simulink model "EPT"  (R2019b)
settings: Solver=FixedStepDiscrete  StartTime=0.0  StopTime=5  FixedStep=0.005  RelTol=1e-3  EnableMultiTasking=on
PreLoadFcn:
  | try, model_open; catch, disp('Error occurred while executing model pre-load callback: model_open.m'); disp('Please assure that the MATLAB working directory is set to the model directory before opening.'); end
InitFcn:
  | try, model_open; catch, end
undefined symbols (not defined in the file or in its folder): Bridge, GCM, H, ln, raptor_get_param_eval, raptor_get_safe_string, raptor_xcp_function
libraries: Raptor_lib x2810, simulink x374, hdlsllib x19
(part 24 of 45)

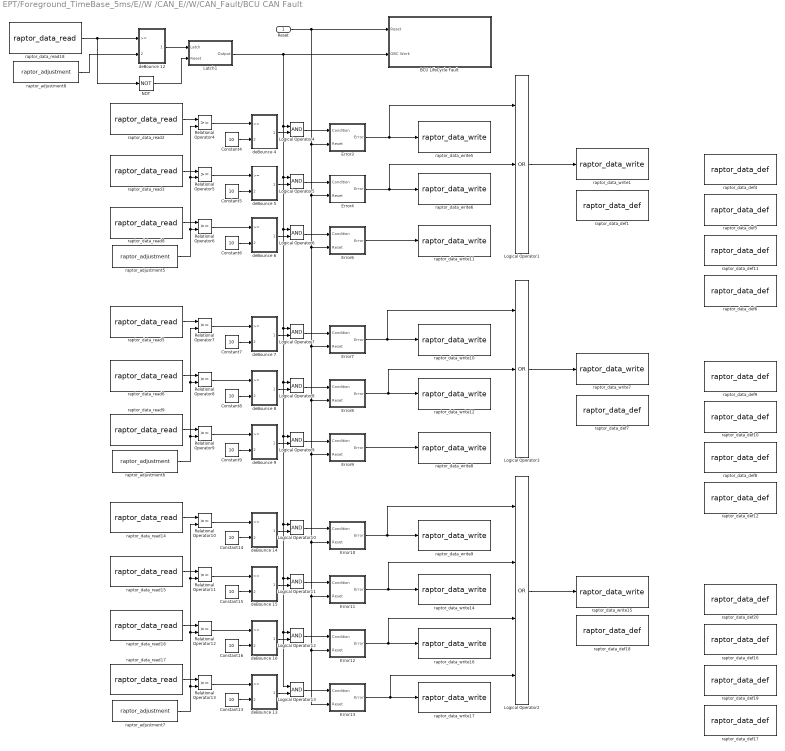
== system EPT/Foreground_TimeBase_5ms/E//W /CAN_E//W/CAN_Fault/BCU CAN Fault ==
  Reset : Inport
  BCU LifeCycle Fault : Subsystem
  Constant{4..9,13..16} (10 alike) : Constant  Value=10
  Error10 : Subsystem
  Error11 : Subsystem
  Error12 : Subsystem
  Error13 : Subsystem
  Error3 : Subsystem
  Error4 : Subsystem
  Error6 : Subsystem
  Error7 : Subsystem
  Error8 : Subsystem
  Error9 : Subsystem
  Latch1 : Subsystem
  Logical Operator1 : Logic  Operator=OR  Inputs=3  AllPortsSameDT=off  OutDataTypeStr=boolean
  Logical Operator{4..13} (10 alike) : Logic  AllPortsSameDT=off  OutDataTypeStr=boolean
  Logical Operator2 : Logic  Operator=OR  Inputs=4  AllPortsSameDT=off  OutDataTypeStr=boolean
  Logical Operator3 : Logic  Operator=OR  Inputs=3  AllPortsSameDT=off  OutDataTypeStr=boolean
  NOT : Logic  Operator=NOT  IconShape=distinctive  AllPortsSameDT=off  OutDataTypeStr=boolean
  Relational Operator{4..13} (10 alike) : RelationalOperator  OutDataTypeStr=boolean  RndMeth=Simplest
  deBounce 12 : Subsystem
  deBounce 13 : Subsystem
  deBounce 14 : Subsystem
  deBounce 15 : Subsystem
  deBounce 16 : Subsystem
  deBounce 4 : Subsystem
  deBounce 5 : Subsystem
  deBounce 6 : Subsystem
  deBounce 7 : Subsystem
  deBounce 8 : Subsystem
  deBounce 9 : Subsystem
  raptor_adjustment5 : Raptor_lib/Data Storage/raptor_adjustment  paramName='CMU1_Age_Time'  nameSource=Parameter  initValue=5  dataType=uint16  storage=Calibration  calDispType=Number  calEnum={'False', 'True'}  calGain=1.0  calOffset=0.0  calMax=inf  calMin=-inf  calFormat='-1'  calUnit=''  calHelp=''  calAccess=1  calFunction=raptor_xcp_function(gcb)  calDispHeaders=off  calColHeaders={'Col1' 'Col2' 'Col3'}  calRowHeaders={'Row1' 'Row2' 'Row3'}
      settings: SourceProductName=Raptor
  raptor_adjustment6 : Raptor_lib/Data Storage/raptor_adjustment  paramName='CMU2_Age_Time'  nameSource=Parameter  initValue=5  dataType=uint16  storage=Calibration  calDispType=Number  calEnum={'False', 'True'}  calGain=1.0  calOffset=0.0  calMax=inf  calMin=-inf  calFormat='-1'  calUnit=''  calHelp=''  calAccess=1  calFunction=raptor_xcp_function(gcb)  calDispHeaders=off  calColHeaders={'Col1' 'Col2' 'Col3'}  calRowHeaders={'Row1' 'Row2' 'Row3'}
      settings: SourceProductName=Raptor
  raptor_adjustment7 : Raptor_lib/Data Storage/raptor_adjustment  paramName='IVT_Age_Time'  nameSource=Parameter  initValue=5  dataType=uint16  storage=Calibration  calDispType=Number  calEnum={'False', 'True'}  calGain=1.0  calOffset=0.0  calMax=inf  calMin=-inf  calFormat='-1'  calUnit=''  calHelp=''  calAccess=1  calFunction=raptor_xcp_function(gcb)  calDispHeaders=off  calColHeaders={'Col1' 'Col2' 'Col3'}  calRowHeaders={'Row1' 'Row2' 'Row3'}
      settings: SourceProductName=Raptor
  raptor_adjustment8 : Raptor_lib/Data Storage/raptor_adjustment  paramName='Cal_BCU_CANFault_TimeCount'  nameSource=Parameter  initValue=300  dataType=double  storage=Calibration  calDispType=Number  calEnum={'False', 'True'}  calGain=1.0  calOffset=0.0  calMax=inf  calMin=-inf  calFormat='-1'  calUnit=''  calHelp=''  calAccess=1  calFunction=raptor_xcp_function(gcb)  calDispHeaders=off  calColHeaders={'Col1' 'Col2' 'Col3'}  calRowHeaders={'Row1' 'Row2' 'Row3'}
      settings: SourceProductName=Raptor
  raptor_data_def1 : Raptor_lib/Data Storage/raptor_data_def  dataName='CAN_Fault_CMU1'  initValue=0  dataType=boolean  storage=Volatile (RAM)  calVisible=on  calType=Measurement  calDispType=Number  calEnum={'False', 'True'}  calGain=1.0  calOffset=0  calMin=-inf  calMax=inf  calFormat='-1'  calUnit=''  calHelp=''  calAccess=1  calFunction=raptor_xcp_function(gcb)  calDispHeaders=off  calColHeaders={'Col1' 'Col2' 'Col3'}  calRowHeaders={'Row1' 'Row2' 'Row3'}
      settings: SourceProductName=Raptor
  raptor_data_def10 : Raptor_lib/Data Storage/raptor_data_def  dataName='CAN_Fault_CMU200B1A2'  initValue=0  dataType=boolean  storage=Volatile (RAM)  calVisible=on  calType=Measurement  calDispType=Number  calEnum={'False', 'True'}  calGain=1.0  calOffset=0  calMin=-inf  calMax=inf  calFormat='-1'  calUnit=''  calHelp=''  calAccess=1  calFunction=raptor_xcp_function(gcb)  calDispHeaders=off  calColHeaders={'Col1' 'Col2' 'Col3'}  calRowHeaders={'Row1' 'Row2' 'Row3'}
      settings: SourceProductName=Raptor
  raptor_data_def11 : Raptor_lib/Data Storage/raptor_data_def  dataName='CAN_Fault_CMU200B2A1'  initValue=0  dataType=boolean  storage=Volatile (RAM)  calVisible=on  calType=Measurement  calDispType=Number  calEnum={'False', 'True'}  calGain=1.0  calOffset=0  calMin=-inf  calMax=inf  calFormat='-1'  calUnit=''  calHelp=''  calAccess=1  calFunction=raptor_xcp_function(gcb)  calDispHeaders=off  calColHeaders={'Col1' 'Col2' 'Col3'}  calRowHeaders={'Row1' 'Row2' 'Row3'}
      settings: SourceProductName=Raptor
  raptor_data_def12 : Raptor_lib/Data Storage/raptor_data_def  dataName='CAN_Fault_CMU200BAA2'  initValue=0  dataType=boolean  storage=Volatile (RAM)  calVisible=on  calType=Measurement  calDispType=Number  calEnum={'False', 'True'}  calGain=1.0  calOffset=0  calMin=-inf  calMax=inf  calFormat='-1'  calUnit=''  calHelp=''  calAccess=1  calFunction=raptor_xcp_function(gcb)  calDispHeaders=off  calColHeaders={'Col1' 'Col2' 'Col3'}  calRowHeaders={'Row1' 'Row2' 'Row3'}
      settings: SourceProductName=Raptor
  raptor_data_def16 : Raptor_lib/Data Storage/raptor_data_def  dataName='CAN_Fault_0x522'  initValue=0  dataType=boolean  storage=Volatile (RAM)  calVisible=on  calType=Measurement  calDispType=Number  calEnum={'False', 'True'}  calGain=1.0  calOffset=0  calMin=-inf  calMax=inf  calFormat='-1'  calUnit=''  calHelp=''  calAccess=1  calFunction=raptor_xcp_function(gcb)  calDispHeaders=off  calColHeaders={'Col1' 'Col2' 'Col3'}  calRowHeaders={'Row1' 'Row2' 'Row3'}
      settings: SourceProductName=Raptor
  raptor_data_def17 : Raptor_lib/Data Storage/raptor_data_def  dataName='CAN_Fault_0x524'  initValue=0  dataType=boolean  storage=Volatile (RAM)  calVisible=on  calType=Measurement  calDispType=Number  calEnum={'False', 'True'}  calGain=1.0  calOffset=0  calMin=-inf  calMax=inf  calFormat='-1'  calUnit=''  calHelp=''  calAccess=1  calFunction=raptor_xcp_function(gcb)  calDispHeaders=off  calColHeaders={'Col1' 'Col2' 'Col3'}  calRowHeaders={'Row1' 'Row2' 'Row3'}
      settings: SourceProductName=Raptor
  raptor_data_def18 : Raptor_lib/Data Storage/raptor_data_def  dataName='CAN_Fault_IVT'  initValue=0  dataType=boolean  storage=Volatile (RAM)  calVisible=on  calType=Measurement  calDispType=Number  calEnum={'False', 'True'}  calGain=1.0  calOffset=0  calMin=-inf  calMax=inf  calFormat='-1'  calUnit=''  calHelp=''  calAccess=1  calFunction=raptor_xcp_function(gcb)  calDispHeaders=off  calColHeaders={'Col1' 'Col2' 'Col3'}  calRowHeaders={'Row1' 'Row2' 'Row3'}
      settings: SourceProductName=Raptor
  raptor_data_def19 : Raptor_lib/Data Storage/raptor_data_def  dataName='CAN_Fault_0x523'  initValue=0  dataType=boolean  storage=Volatile (RAM)  calVisible=on  calType=Measurement  calDispType=Number  calEnum={'False', 'True'}  calGain=1.0  calOffset=0  calMin=-inf  calMax=inf  calFormat='-1'  calUnit=''  calHelp=''  calAccess=1  calFunction=raptor_xcp_function(gcb)  calDispHeaders=off  calColHeaders={'Col1' 'Col2' 'Col3'}  calRowHeaders={'Row1' 'Row2' 'Row3'}
      settings: SourceProductName=Raptor
  raptor_data_def20 : Raptor_lib/Data Storage/raptor_data_def  dataName='CAN_Fault_0x521'  initValue=0  dataType=boolean  storage=Volatile (RAM)  calVisible=on  calType=Measurement  calDispType=Number  calEnum={'False', 'True'}  calGain=1.0  calOffset=0  calMin=-inf  calMax=inf  calFormat='-1'  calUnit=''  calHelp=''  calAccess=1  calFunction=raptor_xcp_function(gcb)  calDispHeaders=off  calColHeaders={'Col1' 'Col2' 'Col3'}  calRowHeaders={'Row1' 'Row2' 'Row3'}
      settings: SourceProductName=Raptor
  raptor_data_def4 : Raptor_lib/Data Storage/raptor_data_def  dataName='CAN_Fault_CMU200B0A1'  initValue=0  dataType=boolean  storage=Volatile (RAM)  calVisible=on  calType=Measurement  calDispType=Number  calEnum={'False', 'True'}  calGain=1.0  calOffset=0  calMin=-inf  calMax=inf  calFormat='-1'  calUnit=''  calHelp=''  calAccess=1  calFunction=raptor_xcp_function(gcb)  calDispHeaders=off  calColHeaders={'Col1' 'Col2' 'Col3'}  calRowHeaders={'Row1' 'Row2' 'Row3'}
      settings: SourceProductName=Raptor
  raptor_data_def5 : Raptor_lib/Data Storage/raptor_data_def  dataName='CAN_Fault_CMU200B1A1'  initValue=0  dataType=boolean  storage=Volatile (RAM)  calVisible=on  calType=Measurement  calDispType=Number  calEnum={'False', 'True'}  calGain=1.0  calOffset=0  calMin=-inf  calMax=inf  calFormat='-1'  calUnit=''  calHelp=''  calAccess=1  calFunction=raptor_xcp_function(gcb)  calDispHeaders=off  calColHeaders={'Col1' 'Col2' 'Col3'}  calRowHeaders={'Row1' 'Row2' 'Row3'}
      settings: SourceProductName=Raptor
  raptor_data_def6 : Raptor_lib/Data Storage/raptor_data_def  dataName='CAN_Fault_CMU200BAA1'  initValue=0  dataType=boolean  storage=Volatile (RAM)  calVisible=on  calType=Measurement  calDispType=Number  calEnum={'False', 'True'}  calGain=1.0  calOffset=0  calMin=-inf  calMax=inf  calFormat='-1'  calUnit=''  calHelp=''  calAccess=1  calFunction=raptor_xcp_function(gcb)  calDispHeaders=off  calColHeaders={'Col1' 'Col2' 'Col3'}  calRowHeaders={'Row1' 'Row2' 'Row3'}
      settings: SourceProductName=Raptor
  raptor_data_def7 : Raptor_lib/Data Storage/raptor_data_def  dataName='CAN_Fault_CMU2'  initValue=0  dataType=boolean  storage=Volatile (RAM)  calVisible=on  calType=Measurement  calDispType=Number  calEnum={'False', 'True'}  calGain=1.0  calOffset=0  calMin=-inf  calMax=inf  calFormat='-1'  calUnit=''  calHelp=''  calAccess=1  calFunction=raptor_xcp_function(gcb)  calDispHeaders=off  calColHeaders={'Col1' 'Col2' 'Col3'}  calRowHeaders={'Row1' 'Row2' 'Row3'}
      settings: SourceProductName=Raptor
  raptor_data_def8 : Raptor_lib/Data Storage/raptor_data_def  dataName='CAN_Fault_CMU200B2A2'  initValue=0  dataType=boolean  storage=Volatile (RAM)  calVisible=on  calType=Measurement  calDispType=Number  calEnum={'False', 'True'}  calGain=1.0  calOffset=0  calMin=-inf  calMax=inf  calFormat='-1'  calUnit=''  calHelp=''  calAccess=1  calFunction=raptor_xcp_function(gcb)  calDispHeaders=off  calColHeaders={'Col1' 'Col2' 'Col3'}  calRowHeaders={'Row1' 'Row2' 'Row3'}
      settings: SourceProductName=Raptor
  raptor_data_def9 : Raptor_lib/Data Storage/raptor_data_def  dataName='CAN_Fault_CMU200B0A2'  initValue=0  dataType=boolean  storage=Volatile (RAM)  calVisible=on  calType=Measurement  calDispType=Number  calEnum={'False', 'True'}  calGain=1.0  calOffset=0  calMin=-inf  calMax=inf  calFormat='-1'  calUnit=''  calHelp=''  calAccess=1  calFunction=raptor_xcp_function(gcb)  calDispHeaders=off  calColHeaders={'Col1' 'Col2' 'Col3'}  calRowHeaders={'Row1' 'Row2' 'Row3'}
      settings: SourceProductName=Raptor
  raptor_data_read14 : Raptor_lib/Data Storage/raptor_data_read  dataName='Age_0x521'  dataShape=Scalar  idxSource=Input  idxRow=1  idxCol=1
      settings: SourceProductName=Raptor
  raptor_data_read15 : Raptor_lib/Data Storage/raptor_data_read  dataName='Age_0x522'  dataShape=Scalar  idxSource=Input  idxRow=1  idxCol=1
      settings: SourceProductName=Raptor
  raptor_data_read16 : Raptor_lib/Data Storage/raptor_data_read  dataName='Age_0x523'  dataShape=Scalar  idxSource=Input  idxRow=1  idxCol=1
      settings: SourceProductName=Raptor
  raptor_data_read17 : Raptor_lib/Data Storage/raptor_data_read  dataName='Age_0x524'  dataShape=Scalar  idxSource=Input  idxRow=1  idxCol=1
      settings: SourceProductName=Raptor
  raptor_data_read18 : Raptor_lib/Data Storage/raptor_data_read  dataName='Relay_BMS_OBU'  dataShape=Scalar  idxSource=Input  idxRow=1  idxCol=1
      settings: SourceProductName=Raptor
  raptor_data_read2 : Raptor_lib/Data Storage/raptor_data_read  dataName='Rx0x200B0A1_Age'  dataShape=Scalar  idxSource=Input  idxRow=1  idxCol=1
      settings: SourceProductName=Raptor
  raptor_data_read3 : Raptor_lib/Data Storage/raptor_data_read  dataName='Rx0x200B1A1_Age'  dataShape=Scalar  idxSource=Input  idxRow=1  idxCol=1
      settings: SourceProductName=Raptor
  raptor_data_read5 : Raptor_lib/Data Storage/raptor_data_read  dataName='Rx0x200B0A2_Age'  dataShape=Scalar  idxSource=Input  idxRow=1  idxCol=1
      settings: SourceProductName=Raptor
  raptor_data_read6 : Raptor_lib/Data Storage/raptor_data_read  dataName='Rx0x200B1A2_Age'  dataShape=Scalar  idxSource=Input  idxRow=1  idxCol=1
      settings: SourceProductName=Raptor
  raptor_data_read8 : Raptor_lib/Data Storage/raptor_data_read  dataName='Rx0x200B2A1_Age'  dataShape=Scalar  idxSource=Input  idxRow=1  idxCol=1
      settings: SourceProductName=Raptor
  raptor_data_read9 : Raptor_lib/Data Storage/raptor_data_read  dataName='Rx0x200B2A2_Age'  dataShape=Scalar  idxSource=Input  idxRow=1  idxCol=1
      settings: SourceProductName=Raptor
  raptor_data_write1 : Raptor_lib/Data Storage/raptor_data_write  dataName='CAN_Fault_CMU1'  dataShape=Scalar  idxSource=Input Port  idxRow=1  idxCol=1
      settings: SourceProductName=Raptor
  raptor_data_write10 : Raptor_lib/Data Storage/raptor_data_write  dataName='CAN_Fault_CMU200B0A2'  dataShape=Scalar  idxSource=Input Port  idxRow=1  idxCol=1
      settings: SourceProductName=Raptor
  raptor_data_write11 : Raptor_lib/Data Storage/raptor_data_write  dataName='CAN_Fault_CMU200B2A1'  dataShape=Scalar  idxSource=Input Port  idxRow=1  idxCol=1
      settings: SourceProductName=Raptor
  raptor_data_write12 : Raptor_lib/Data Storage/raptor_data_write  dataName='CAN_Fault_CMU200B1A2'  dataShape=Scalar  idxSource=Input Port  idxRow=1  idxCol=1
      settings: SourceProductName=Raptor
  raptor_data_write14 : Raptor_lib/Data Storage/raptor_data_write  dataName='CAN_Fault_0x522'  dataShape=Scalar  idxSource=Input Port  idxRow=1  idxCol=1
      settings: SourceProductName=Raptor
  raptor_data_write15 : Raptor_lib/Data Storage/raptor_data_write  dataName='CAN_Fault_IVT'  dataShape=Scalar  idxSource=Input Port  idxRow=1  idxCol=1
      settings: SourceProductName=Raptor
  raptor_data_write16 : Raptor_lib/Data Storage/raptor_data_write  dataName='CAN_Fault_0x523'  dataShape=Scalar  idxSource=Input Port  idxRow=1  idxCol=1
      settings: SourceProductName=Raptor
  raptor_data_write17 : Raptor_lib/Data Storage/raptor_data_write  dataName='CAN_Fault_0x524'  dataShape=Scalar  idxSource=Input Port  idxRow=1  idxCol=1
      settings: SourceProductName=Raptor
  raptor_data_write5 : Raptor_lib/Data Storage/raptor_data_write  dataName='CAN_Fault_CMU200B0A1'  dataShape=Scalar  idxSource=Input Port  idxRow=1  idxCol=1
      settings: SourceProductName=Raptor
  raptor_data_write6 : Raptor_lib/Data Storage/raptor_data_write  dataName='CAN_Fault_CMU200B1A1'  dataShape=Scalar  idxSource=Input Port  idxRow=1  idxCol=1
      settings: SourceProductName=Raptor
  raptor_data_write7 : Raptor_lib/Data Storage/raptor_data_write  dataName='CAN_Fault_CMU2'  dataShape=Scalar  idxSource=Input Port  idxRow=1  idxCol=1
      settings: SourceProductName=Raptor
  raptor_data_write8 : Raptor_lib/Data Storage/raptor_data_write  dataName='CAN_Fault_CMU200B2A2'  dataShape=Scalar  idxSource=Input Port  idxRow=1  idxCol=1
      settings: SourceProductName=Raptor
  raptor_data_write9 : Raptor_lib/Data Storage/raptor_data_write  dataName='CAN_Fault_0x521'  dataShape=Scalar  idxSource=Input Port  idxRow=1  idxCol=1
      settings: SourceProductName=Raptor
  wires:
  Error10/1(Error) -> raptor_data_write9/1, Logical Operator2/1
  raptor_data_read16/1 -> Relational Operator12/1
  raptor_data_read15/1 -> Relational Operator11/1
  raptor_data_read8/1 -> Relational Operator6/1
  Constant8/1 -> deBounce 8/2(TimeCount1)
  Error7/1(Error) -> Logical Operator3/1, raptor_data_write10/1
  Error8/1(Error) -> raptor_data_write12/1, Logical Operator3/2
  Error13/1(Error) -> Logical Operator2/4, raptor_data_write17/1
  raptor_data_read3/1 -> Relational Operator5/1
  Error9/1(Error) -> raptor_data_write8/1
  Logical Operator3/1 -> raptor_data_write7/1
  Relational Operator13/1 -> deBounce 13/1(>=)
  raptor_data_read6/1 -> Relational Operator8/1
  Relational Operator5/1 -> deBounce 5/1(>=)
  Error4/1(Error) -> raptor_data_write6/1, Logical Operator1/2
  Relational Operator12/1 -> deBounce 16/1(>=)
  raptor_adjustment6/1 -> Relational Operator9/2, Relational Operator8/2, Relational Operator7/2
  Constant7/1 -> deBounce 7/2(TimeCount1)
  Constant6/1 -> deBounce 6/2(TimeCount1)
  Relational Operator8/1 -> deBounce 8/1(>=)
  Relational Operator10/1 -> deBounce 14/1(>=)
  Constant4/1 -> deBounce 4/2(TimeCount1)
  Error6/1(Error) -> raptor_data_write11/1
  raptor_adjustment8/1 -> deBounce 12/2(TimeCount1)
  Relational Operator7/1 -> deBounce 7/1(>=)
  Relational Operator9/1 -> deBounce 9/1(>=)
  raptor_data_read5/1 -> Relational Operator7/1
  Relational Operator11/1 -> deBounce 15/1(>=)
  raptor_adjustment5/1 -> Relational Operator4/2, Relational Operator5/2, Relational Operator6/2
  Constant16/1 -> deBounce 16/2(TimeCount1)
  Constant5/1 -> deBounce 5/2(TimeCount1)
  Error12/1(Error) -> raptor_data_write16/1, Logical Operator2/3
  raptor_data_read2/1 -> Relational Operator4/1
  Error3/1(Error) -> Logical Operator1/1, raptor_data_write5/1
  Constant14/1 -> deBounce 14/2(TimeCount1)
  Error11/1(Error) -> Logical Operator2/2, raptor_data_write14/1
  raptor_data_read14/1 -> Relational Operator10/1
  Logical Operator1/1 -> raptor_data_write1/1
  raptor_data_read9/1 -> Relational Operator9/1
  Relational Operator4/1 -> deBounce 4/1(>=)
  Relational Operator6/1 -> deBounce 6/1(>=)
  Logical Operator2/1 -> raptor_data_write15/1
  Constant13/1 -> deBounce 13/2(TimeCount1)
  Constant15/1 -> deBounce 15/2(TimeCount1)
  Constant9/1 -> deBounce 9/2(TimeCount1)
  raptor_adjustment7/1 -> Relational Operator13/2, Relational Operator12/2, Relational Operator11/2, Relational Operator10/2
  raptor_data_read17/1 -> Relational Operator13/1
  deBounce 4/1(Tirgger1) -> Logical Operator4/2
  Logical Operator4/1 -> Error3/1(Condition)
  deBounce 5/1(Tirgger1) -> Logical Operator5/2
  Logical Operator5/1 -> Error4/1(Condition)
  deBounce 6/1(Tirgger1) -> Logical Operator6/2
  Logical Operator6/1 -> Error6/1(Condition)
  Logical Operator7/1 -> Error7/1(Condition)
  deBounce 7/1(Tirgger1) -> Logical Operator7/2
  deBounce 8/1(Tirgger1) -> Logical Operator8/2
  Logical Operator8/1 -> Error8/1(Condition)
  deBounce 9/1(Tirgger1) -> Logical Operator9/2
  Logical Operator9/1 -> Error9/1(Condition)
  deBounce 14/1(Tirgger1) -> Logical Operator10/2
  Logical Operator10/1 -> Error10/1(Condition)
  deBounce 15/1(Tirgger1) -> Logical Operator11/2
  Logical Operator11/1 -> Error11/1(Condition)
  deBounce 16/1(Tirgger1) -> Logical Operator12/2
  Logical Operator12/1 -> Error12/1(Condition)
  deBounce 13/1(Tirgger1) -> Logical Operator13/2
  Logical Operator13/1 -> Error13/1(Condition)
  NOT/1 -> Latch1/2(Reset)
  raptor_data_read18/1 -> NOT/1, deBounce 12/1(>=)
  deBounce 12/1(Tirgger1) -> Latch1/1(Latch)
  Latch1/1(Output) -> Logical Operator13/1, Logical Operator12/1, Logical Operator11/1, Logical Operator10/1, Logical Operator9/1, Logical Operator8/1, Logical Operator7/1, Logical Operator6/1, Logical Operator5/1, Logical Operator4/1, BCU LifeCycle Fault/2(OBC Work)
  Reset/1 -> Error13/2(Reset), Error12/2(Reset), Error11/2(Reset), Error10/2(Reset), Error9/2(Reset), Error8/2(Reset), Error7/2(Reset), Error6/2(Reset), Error4/2(Reset), Error3/2(Reset), BCU LifeCycle Fault/1(Reset)

== system EPT/Foreground_TimeBase_5ms/E//W /CAN_E//W/CAN_Fault/DCDC CAN Fault ==
  Reset : Inport
  Constant1 : Constant  Value=10
  Latch1 : Subsystem
  Latch2 : Subsystem
  Logical Operator4 : Logic  AllPortsSameDT=off  OutDataTypeStr=boolean
  NOT : Logic  Operator=NOT  IconShape=distinctive  AllPortsSameDT=off  OutDataTypeStr=boolean
  Relational Operator : RelationalOperator  OutDataTypeStr=boolean  RndMeth=Simplest
  deBounce 1 : Subsystem
  deBounce 10 : Subsystem
  raptor_adjustment6 : Raptor_lib/Data Storage/raptor_adjustment  paramName='DCDC_Age_Time'  nameSource=Parameter  initValue=5  dataType=uint16  storage=Calibration  calDispType=Number  calEnum={'False', 'True'}  calGain=1.0  calOffset=0.0  calMax=inf  calMin=-inf  calFormat='-1'  calUnit=''  calHelp=''  calAccess=1  calFunction=raptor_xcp_function(gcb)  calDispHeaders=off  calColHeaders={'Col1' 'Col2' 'Col3'}  calRowHeaders={'Row1' 'Row2' 'Row3'}
      settings: SourceProductName=Raptor
  raptor_adjustment8 : Raptor_lib/Data Storage/raptor_adjustment  paramName='Cal_DCDC_CANFault_TimeCount'  nameSource=Parameter  initValue=250  dataType=double  storage=Calibration  calDispType=Number  calEnum={'False', 'True'}  calGain=1.0  calOffset=0.0  calMax=inf  calMin=-inf  calFormat='-1'  calUnit=''  calHelp=''  calAccess=1  calFunction=raptor_xcp_function(gcb)  calDispHeaders=off  calColHeaders={'Col1' 'Col2' 'Col3'}  calRowHeaders={'Row1' 'Row2' 'Row3'}
      settings: SourceProductName=Raptor
  raptor_data_def : Raptor_lib/Data Storage/raptor_data_def  dataName='CAN_Fault_DCDC'  initValue=0  dataType=boolean  storage=Volatile (RAM)  calVisible=on  calType=Measurement  calDispType=Number  calEnum={'False', 'True'}  calGain=1.0  calOffset=0  calMin=-inf  calMax=inf  calFormat='-1'  calUnit=''  calHelp=''  calAccess=1  calFunction=raptor_xcp_function(gcb)  calDispHeaders=off  calColHeaders={'Col1' 'Col2' 'Col3'}  calRowHeaders={'Row1' 'Row2' 'Row3'}
      settings: SourceProductName=Raptor
  raptor_data_read : Raptor_lib/Data Storage/raptor_data_read  dataName='Rx0x180XF4D5_Age'  dataShape=Scalar  idxSource=Input  idxRow=1  idxCol=1
      settings: SourceProductName=Raptor
  raptor_data_read7 : Raptor_lib/Data Storage/raptor_data_read  dataName='Relay_DCDC_12V'  dataShape=Scalar  idxSource=Input  idxRow=1  idxCol=1
      settings: SourceProductName=Raptor
  raptor_data_write2 : Raptor_lib/Data Storage/raptor_data_write  dataName='CAN_Fault_DCDC'  dataShape=Scalar  idxSource=Input Port  idxRow=1  idxCol=1
      settings: SourceProductName=Raptor
  wires:
  Reset/1 -> Latch2/2(Reset)
  NOT/1 -> Latch1/2(Reset)
  raptor_data_read/1 -> Relational Operator/1
  raptor_adjustment8/1 -> deBounce 10/2(TimeCount1)
  deBounce 10/1(Tirgger1) -> Latch1/1(Latch)
  Latch2/1(Output) -> raptor_data_write2/1
  Logical Operator4/1 -> Latch2/1(Latch)
  Constant1/1 -> deBounce 1/2(TimeCount1)
  deBounce 1/1(Tirgger1) -> Logical Operator4/2
  raptor_data_read7/1 -> deBounce 10/1(>=), NOT/1
  Relational Operator/1 -> deBounce 1/1(>=)
  Latch1/1(Output) -> Logical Operator4/1
  raptor_adjustment6/1 -> Relational Operator/2

== system EPT/Foreground_TimeBase_5ms/E//W /CAN_E//W/CAN_Fault/ECHS CAN Fault ==
  Reset : Inport
  Constant : Constant  Value=10
  Latch1 : Subsystem
  Latch5 : Subsystem
  Logical Operator4 : Logic  AllPortsSameDT=off  OutDataTypeStr=boolean
  Relational Operator3 : RelationalOperator  OutDataTypeStr=boolean  RndMeth=Simplest
  "deBounce " : Subsystem
  deBounce 1 : Subsystem
  raptor_adjustment1 : Raptor_lib/Data Storage/raptor_adjustment  paramName='Cal_ECHS_CANFault_TimeCount'  nameSource=Parameter  initValue=200  dataType=double  storage=Calibration  calDispType=Number  calEnum={'False', 'True'}  calGain=1.0  calOffset=0.0  calMax=inf  calMin=-inf  calFormat='-1'  calUnit=''  calHelp=''  calAccess=1  calFunction=raptor_xcp_function(gcb)  calDispHeaders=off  calColHeaders={'Col1' 'Col2' 'Col3'}  calRowHeaders={'Row1' 'Row2' 'Row3'}
      settings: SourceProductName=Raptor
  raptor_adjustment4 : Raptor_lib/Data Storage/raptor_adjustment  paramName='Cal_ECHS_Age_Times'  nameSource=Parameter  initValue=10  dataType=uint16  storage=Calibration  calDispType=Number  calEnum={'False', 'True'}  calGain=1.0  calOffset=0.0  calMax=inf  calMin=-inf  calFormat='-1'  calUnit=''  calHelp=''  calAccess=1  calFunction=raptor_xcp_function(gcb)  calDispHeaders=off  calColHeaders={'Col1' 'Col2' 'Col3'}  calRowHeaders={'Row1' 'Row2' 'Row3'}
      settings: SourceProductName=Raptor
  raptor_data_def14 : Raptor_lib/Data Storage/raptor_data_def  dataName='Flag_ECHS_Disconnected'  initValue=0  dataType=boolean  storage=Volatile (RAM)  calVisible=on  calType=Measurement  calDispType=Number  calEnum={'False', 'True'}  calGain=1.0  calOffset=0  calMin=-inf  calMax=inf  calFormat='-1'  calUnit=''  calHelp=''  calAccess=1  calFunction=raptor_xcp_function(gcb)  calDispHeaders=off  calColHeaders={'Col1' 'Col2' 'Col3'}  calRowHeaders={'Row1' 'Row2' 'Row3'}
      settings: SourceProductName=Raptor
  raptor_data_read12 : Raptor_lib/Data Storage/raptor_data_read  dataName='Rx0xC10F4D0_Age'  dataShape=Scalar  idxSource=Input  idxRow=1  idxCol=1
      settings: SourceProductName=Raptor
  raptor_data_read4 : Raptor_lib/Data Storage/raptor_data_read  dataName='Flag_ECHS_CAN_Work'  dataShape=Scalar  idxSource=Input  idxRow=1  idxCol=1
      settings: SourceProductName=Raptor
  raptor_data_write4 : Raptor_lib/Data Storage/raptor_data_write  dataName='Flag_ECHS_Disconnected'  dataShape=Scalar  idxSource=Input Port  idxRow=1  idxCol=1
      settings: SourceProductName=Raptor
  wires:
  Relational Operator3/1 -> "deBounce "/1(>=)
  Constant/1 -> "deBounce "/2(TimeCount1)
  Reset/1 -> Latch1/2(Reset), Latch5/2(Reset)
  "deBounce "/1(Tirgger1) -> Logical Operator4/2
  raptor_data_read4/1 -> deBounce 1/1(>=)
  raptor_adjustment4/1 -> Relational Operator3/2
  Latch5/1(Output) -> raptor_data_write4/1
  raptor_data_read12/1 -> Relational Operator3/1
  raptor_adjustment1/1 -> deBounce 1/2(TimeCount1)
  Logical Operator4/1 -> Latch5/1(Latch)
  deBounce 1/1(Tirgger1) -> Latch1/1(Latch)
  Latch1/1(Output) -> Logical Operator4/1

== system EPT/Foreground_TimeBase_5ms/E//W /CAN_E//W/CAN_Fault/MCU CAN Fault ==
  Reset : Inport
  Constant1 : Constant  Value=10
  Constant2 : Constant  Value=10
  Constant3 : Constant  Value=10
  Latch1 : Subsystem
  Latch2 : Subsystem
  Latch3 : Subsystem
  Latch4 : Subsystem
  Logical Operator : Logic  Operator=OR  Inputs=3  AllPortsSameDT=off  OutDataTypeStr=boolean
  Logical Operator4 : Logic  AllPortsSameDT=off  OutDataTypeStr=boolean
  Logical Operator5 : Logic  AllPortsSameDT=off  OutDataTypeStr=boolean
  Logical Operator6 : Logic  AllPortsSameDT=off  OutDataTypeStr=boolean
  NOT : Logic  Operator=NOT  IconShape=distinctive  AllPortsSameDT=off  OutDataTypeStr=boolean
  Relational Operator : RelationalOperator  OutDataTypeStr=boolean  RndMeth=Simplest
  Relational Operator1 : RelationalOperator  OutDataTypeStr=boolean  RndMeth=Simplest
  Relational Operator2 : RelationalOperator  OutDataTypeStr=boolean  RndMeth=Simplest
  deBounce 1 : Subsystem
  deBounce 10 : Subsystem
  deBounce 2 : Subsystem
  deBounce 3 : Subsystem
  raptor_adjustment3 : Raptor_lib/Data Storage/raptor_adjustment  paramName='MCU_Age_Times'  nameSource=Parameter  initValue=10  dataType=uint16  storage=Calibration  calDispType=Number  calEnum={'False', 'True'}  calGain=1.0  calOffset=0.0  calMax=inf  calMin=-inf  calFormat='-1'  calUnit=''  calHelp=''  calAccess=1  calFunction=raptor_xcp_function(gcb)  calDispHeaders=off  calColHeaders={'Col1' 'Col2' 'Col3'}  calRowHeaders={'Row1' 'Row2' 'Row3'}
      settings: SourceProductName=Raptor
  raptor_adjustment8 : Raptor_lib/Data Storage/raptor_adjustment  paramName='Cal_MCU_CANFault_TimeCount'  nameSource=Parameter  initValue=300  dataType=double  storage=Calibration  calDispType=Number  calEnum={'False', 'True'}  calGain=1.0  calOffset=0.0  calMax=inf  calMin=-inf  calFormat='-1'  calUnit=''  calHelp=''  calAccess=1  calFunction=raptor_xcp_function(gcb)  calDispHeaders=off  calColHeaders={'Col1' 'Col2' 'Col3'}  calRowHeaders={'Row1' 'Row2' 'Row3'}
      settings: SourceProductName=Raptor
  raptor_data_def : Raptor_lib/Data Storage/raptor_data_def  dataName='CAN_Fault_MCU'  initValue=0  dataType=boolean  storage=Volatile (RAM)  calVisible=on  calType=Measurement  calDispType=Number  calEnum={'False', 'True'}  calGain=1.0  calOffset=0  calMin=-inf  calMax=inf  calFormat='-1'  calUnit=''  calHelp=''  calAccess=1  calFunction=raptor_xcp_function(gcb)  calDispHeaders=off  calColHeaders={'Col1' 'Col2' 'Col3'}  calRowHeaders={'Row1' 'Row2' 'Row3'}
      settings: SourceProductName=Raptor
  raptor_data_def13 : Raptor_lib/Data Storage/raptor_data_def  dataName='CAN_Fault_MCU0x220'  initValue=0  dataType=boolean  storage=Volatile (RAM)  calVisible=on  calType=Measurement  calDispType=Number  calEnum={'False', 'True'}  calGain=1.0  calOffset=0  calMin=-inf  calMax=inf  calFormat='-1'  calUnit=''  calHelp=''  calAccess=1  calFunction=raptor_xcp_function(gcb)  calDispHeaders=off  calColHeaders={'Col1' 'Col2' 'Col3'}  calRowHeaders={'Row1' 'Row2' 'Row3'}
      settings: SourceProductName=Raptor
  raptor_data_def2 : Raptor_lib/Data Storage/raptor_data_def  dataName='CAN_Fault_MCU0x221'  initValue=0  dataType=boolean  storage=Volatile (RAM)  calVisible=on  calType=Measurement  calDispType=Number  calEnum={'False', 'True'}  calGain=1.0  calOffset=0  calMin=-inf  calMax=inf  calFormat='-1'  calUnit=''  calHelp=''  calAccess=1  calFunction=raptor_xcp_function(gcb)  calDispHeaders=off  calColHeaders={'Col1' 'Col2' 'Col3'}  calRowHeaders={'Row1' 'Row2' 'Row3'}
      settings: SourceProductName=Raptor
  raptor_data_def3 : Raptor_lib/Data Storage/raptor_data_def  dataName='CAN_Fault_MCU0x701'  initValue=0  dataType=boolean  storage=Volatile (RAM)  calVisible=on  calType=Measurement  calDispType=Number  calEnum={'False', 'True'}  calGain=1.0  calOffset=0  calMin=-inf  calMax=inf  calFormat='-1'  calUnit=''  calHelp=''  calAccess=1  calFunction=raptor_xcp_function(gcb)  calDispHeaders=off  calColHeaders={'Col1' 'Col2' 'Col3'}  calRowHeaders={'Row1' 'Row2' 'Row3'}
      settings: SourceProductName=Raptor
  raptor_data_read : Raptor_lib/Data Storage/raptor_data_read  dataName='Rx0x220_Age'  dataShape=Scalar  idxSource=Input  idxRow=1  idxCol=1
      settings: SourceProductName=Raptor
  raptor_data_read1 : Raptor_lib/Data Storage/raptor_data_read  dataName='Rx0x221_Age'  dataShape=Scalar  idxSource=Input  idxRow=1  idxCol=1
      settings: SourceProductName=Raptor
  raptor_data_read11 : Raptor_lib/Data Storage/raptor_data_read  dataName='Rx0x701_Age'  dataShape=Scalar  idxSource=Input  idxRow=1  idxCol=1
      settings: SourceProductName=Raptor
  raptor_data_read7 : Raptor_lib/Data Storage/raptor_data_read  dataName='Relay_MCU'  dataShape=Scalar  idxSource=Input  idxRow=1  idxCol=1
      settings: SourceProductName=Raptor
  raptor_data_write : Raptor_lib/Data Storage/raptor_data_write  dataName='CAN_Fault_MCU'  dataShape=Scalar  idxSource=Input Port  idxRow=1  idxCol=1
      settings: SourceProductName=Raptor
  raptor_data_write13 : Raptor_lib/Data Storage/raptor_data_write  dataName='CAN_Fault_MCU0x701'  dataShape=Scalar  idxSource=Input Port  idxRow=1  idxCol=1
      settings: SourceProductName=Raptor
  raptor_data_write2 : Raptor_lib/Data Storage/raptor_data_write  dataName='CAN_Fault_MCU0x220'  dataShape=Scalar  idxSource=Input Port  idxRow=1  idxCol=1
      settings: SourceProductName=Raptor
  raptor_data_write3 : Raptor_lib/Data Storage/raptor_data_write  dataName='CAN_Fault_MCU0x221'  dataShape=Scalar  idxSource=Input Port  idxRow=1  idxCol=1
      settings: SourceProductName=Raptor
  wires:
  Latch1/1(Output) -> Logical Operator6/1, Logical Operator5/1, Logical Operator4/1
  Relational Operator/1 -> deBounce 1/1(>=)
  Constant3/1 -> deBounce 3/2(TimeCount1)
  raptor_data_read1/1 -> Relational Operator1/1
  Constant2/1 -> deBounce 2/2(TimeCount1)
  Relational Operator2/1 -> deBounce 3/1(>=)
  raptor_data_read7/1 -> NOT/1, deBounce 10/1(>=)
  deBounce 3/1(Tirgger1) -> Logical Operator6/2
  raptor_adjustment3/1 -> Relational Operator/2, Relational Operator1/2, Relational Operator2/2
  Relational Operator1/1 -> deBounce 2/1(>=)
  deBounce 1/1(Tirgger1) -> Logical Operator4/2
  Constant1/1 -> deBounce 1/2(TimeCount1)
  Logical Operator4/1 -> Latch2/1(Latch)
  raptor_data_read11/1 -> Relational Operator2/1
  Latch2/1(Output) -> raptor_data_write2/1, Logical Operator/1
  Logical Operator/1 -> raptor_data_write/1
  Logical Operator5/1 -> Latch3/1(Latch)
  Logical Operator6/1 -> Latch4/1(Latch)
  deBounce 10/1(Tirgger1) -> Latch1/1(Latch)
  raptor_adjustment8/1 -> deBounce 10/2(TimeCount1)
  Latch3/1(Output) -> raptor_data_write3/1, Logical Operator/2
  Latch4/1(Output) -> raptor_data_write13/1, Logical Operator/3
  raptor_data_read/1 -> Relational Operator/1
  NOT/1 -> Latch1/2(Reset)
  deBounce 2/1(Tirgger1) -> Logical Operator5/2
  Reset/1 -> Latch4/2(Reset), Latch3/2(Reset), Latch2/2(Reset)

== system EPT/Foreground_TimeBase_5ms/E//W /CAN_E//W/CAN_Fault/OBC CAN Fault ==
  Reset : Inport
  Constant1 : Constant  Value=10
  Latch1 : Subsystem
  Latch2 : Subsystem
  Logical Operator4 : Logic  AllPortsSameDT=off  OutDataTypeStr=boolean
  NOT : Logic  Operator=NOT  IconShape=distinctive  AllPortsSameDT=off  OutDataTypeStr=boolean
  Relational Operator : RelationalOperator  OutDataTypeStr=boolean  RndMeth=Simplest
  "deBounce 1 " : Subsystem
  deBounce 2 : Subsystem
  raptor_adjustment6 : Raptor_lib/Data Storage/raptor_adjustment  paramName='Cal_OBC_Age_Time'  nameSource=Parameter  initValue=5  dataType=uint16  storage=Calibration  calDispType=Number  calEnum={'False', 'True'}  calGain=1.0  calOffset=0.0  calMax=inf  calMin=-inf  calFormat='-1'  calUnit=''  calHelp=''  calAccess=1  calFunction=raptor_xcp_function(gcb)  calDispHeaders=off  calColHeaders={'Col1' 'Col2' 'Col3'}  calRowHeaders={'Row1' 'Row2' 'Row3'}
      settings: SourceProductName=Raptor
  raptor_adjustment8 : Raptor_lib/Data Storage/raptor_adjustment  paramName='Cal_OBC_CANFault_TimeCount'  nameSource=Parameter  initValue=300  dataType=double  storage=Calibration  calDispType=Number  calEnum={'False', 'True'}  calGain=1.0  calOffset=0.0  calMax=inf  calMin=-inf  calFormat='-1'  calUnit=''  calHelp=''  calAccess=1  calFunction=raptor_xcp_function(gcb)  calDispHeaders=off  calColHeaders={'Col1' 'Col2' 'Col3'}  calRowHeaders={'Row1' 'Row2' 'Row3'}
      settings: SourceProductName=Raptor
  raptor_data_def : Raptor_lib/Data Storage/raptor_data_def  dataName='CAN_Fault_OBC'  initValue=0  dataType=boolean  storage=Volatile (RAM)  calVisible=on  calType=Measurement  calDispType=Number  calEnum={'False', 'True'}  calGain=1.0  calOffset=0  calMin=-inf  calMax=inf  calFormat='-1'  calUnit=''  calHelp=''  calAccess=1  calFunction=raptor_xcp_function(gcb)  calDispHeaders=off  calColHeaders={'Col1' 'Col2' 'Col3'}  calRowHeaders={'Row1' 'Row2' 'Row3'}
      settings: SourceProductName=Raptor
  raptor_data_read : Raptor_lib/Data Storage/raptor_data_read  dataName='OBC_Age'  dataShape=Scalar  idxSource=Input  idxRow=1  idxCol=1
      settings: SourceProductName=Raptor
  raptor_data_read7 : Raptor_lib/Data Storage/raptor_data_read  dataName='Relay_CHG_OBC'  dataShape=Scalar  idxSource=Input  idxRow=1  idxCol=1
      settings: SourceProductName=Raptor
  raptor_data_write2 : Raptor_lib/Data Storage/raptor_data_write  dataName='CAN_Fault_OBC'  dataShape=Scalar  idxSource=Input Port  idxRow=1  idxCol=1
      settings: SourceProductName=Raptor
  wires:
  raptor_adjustment6/1 -> Relational Operator/2
  Latch1/1(Output) -> Logical Operator4/1
  Relational Operator/1 -> deBounce 2/1(>=)
  raptor_data_read7/1 -> NOT/1, "deBounce 1 "/1(>=)
  deBounce 2/1(Tirgger1) -> Logical Operator4/2
  Constant1/1 -> deBounce 2/2(TimeCount1)
  Logical Operator4/1 -> Latch2/1(Latch)
  Latch2/1(Output) -> raptor_data_write2/1
  "deBounce 1 "/1(Tirgger1) -> Latch1/1(Latch)
  raptor_adjustment8/1 -> "deBounce 1 "/2(TimeCount1)
  raptor_data_read/1 -> Relational Operator/1
  NOT/1 -> Latch1/2(Reset)
  Reset/1 -> Latch2/2(Reset)

== system EPT/Foreground_TimeBase_5ms/E//W /CAN_E//W/CAN_Fault/Reset Trigger ==
  Reset Trigger : Inport
  Enable : EnablePort
  raptor_data_write9 : Raptor_lib/Data Storage/raptor_data_write  dataName='Fault_Reset_Trigger'  dataShape=Scalar  idxSource=Input Port  idxRow=1  idxCol=1
      settings: SourceProductName=Raptor
  wires:
  Reset Trigger/1 -> raptor_data_write9/1

== system EPT/Foreground_TimeBase_5ms/Oil//Water//Pack Cooling System/AirC1/Delay1/CycleTrigger ==
  In1 : Inport
  In2 : Inport  Port=2
  Add : Sum
  Add1 : Sum
  Add2 : Sum  Inputs=+-
  Constant1 : Constant
  Constant2 : Constant  Value=0
  Constant3 : Constant
  Data Type Conversion1 : DataTypeConversion
  Data Type Conversion2 : DataTypeConversion
  Display : Display
  Relational Operator1 : RelationalOperator  OutDataTypeStr=boolean  RndMeth=Simplest
  Saturation : Saturate  UpperLimit=inf  LowerLimit=2
  Scope : Scope
  Scope1 : Scope
  Scope2 : Scope
  Switch : Switch  Threshold=1
  Unit Delay : UnitDelay  SampleTime=-1  HasFrameUpgradeWarning=on
  Unit Delay1 : UnitDelay  SampleTime=-1  HasFrameUpgradeWarning=on
  Trigger : Outport  VectorParamsAs1DForOutWhenUnconnected=off
  wires:
  Saturation/1 -> Add2/1
  Add/1 -> Switch/1
  In1/1 -> Data Type Conversion2/1
  Unit Delay/1 -> Add/1
  Switch/1 -> Relational Operator1/1, Scope1/1, Unit Delay/1
  Add1/1 -> Scope/1, Unit Delay1/1, Display/1
  Unit Delay1/1 -> Add1/1
  Constant1/1 -> Add1/2
  Relational Operator1/1 -> Scope2/1, Trigger/1
  Data Type Conversion1/1 -> Relational Operator1/2
  Constant2/1 -> Switch/3
  Data Type Conversion2/1 -> Add/2, Switch/2
  Add2/1 -> Data Type Conversion1/1
  In2/1 -> Saturation/1
  Constant3/1 -> Add2/2

== system EPT/Foreground_TimeBase_5ms/Oil//Water//Pack Cooling System/AirC1/Delay2/CycleTrigger ==
  In1 : Inport
  In2 : Inport  Port=2
  Add : Sum
  Add1 : Sum
  Add2 : Sum  Inputs=+-
  Constant1 : Constant
  Constant2 : Constant  Value=0
  Constant3 : Constant
  Data Type Conversion1 : DataTypeConversion
  Data Type Conversion2 : DataTypeConversion
  Display : Display
  Relational Operator1 : RelationalOperator  OutDataTypeStr=boolean  RndMeth=Simplest
  Saturation : Saturate  UpperLimit=inf  LowerLimit=2
  Scope : Scope
  Scope1 : Scope
  Scope2 : Scope
  Switch : Switch  Threshold=1
  Unit Delay : UnitDelay  SampleTime=-1  HasFrameUpgradeWarning=on
  Unit Delay1 : UnitDelay  SampleTime=-1  HasFrameUpgradeWarning=on
  Trigger : Outport  VectorParamsAs1DForOutWhenUnconnected=off
  wires:
  Saturation/1 -> Add2/1
  Add/1 -> Switch/1
  In1/1 -> Data Type Conversion2/1
  Unit Delay/1 -> Add/1
  Switch/1 -> Relational Operator1/1, Scope1/1, Unit Delay/1
  Add1/1 -> Scope/1, Unit Delay1/1, Display/1
  Unit Delay1/1 -> Add1/1
  Constant1/1 -> Add1/2
  Relational Operator1/1 -> Scope2/1, Trigger/1
  Data Type Conversion1/1 -> Relational Operator1/2
  Constant2/1 -> Switch/3
  Data Type Conversion2/1 -> Add/2, Switch/2
  Add2/1 -> Data Type Conversion1/1
  In2/1 -> Saturation/1
  Constant3/1 -> Add2/2

== system EPT/Foreground_TimeBase_5ms/Oil//Water//Pack Cooling System/AirC1/Delay3/CycleTrigger ==
  In1 : Inport
  In2 : Inport  Port=2
  Add : Sum
  Add1 : Sum
  Add2 : Sum  Inputs=+-
  Constant1 : Constant
  Constant2 : Constant  Value=0
  Constant3 : Constant
  Data Type Conversion1 : DataTypeConversion
  Data Type Conversion2 : DataTypeConversion
  Display : Display
  Relational Operator1 : RelationalOperator  OutDataTypeStr=boolean  RndMeth=Simplest
  Saturation : Saturate  UpperLimit=inf  LowerLimit=2
  Scope : Scope
  Scope1 : Scope
  Scope2 : Scope
  Switch : Switch  Threshold=1
  Unit Delay : UnitDelay  SampleTime=-1  HasFrameUpgradeWarning=on
  Unit Delay1 : UnitDelay  SampleTime=-1  HasFrameUpgradeWarning=on
  Trigger : Outport  VectorParamsAs1DForOutWhenUnconnected=off
  wires:
  Constant3/1 -> Add2/2
  In2/1 -> Saturation/1
  Add2/1 -> Data Type Conversion1/1
  Data Type Conversion2/1 -> Switch/2, Add/2
  Constant2/1 -> Switch/3
  Data Type Conversion1/1 -> Relational Operator1/2
  Relational Operator1/1 -> Trigger/1, Scope2/1
  Constant1/1 -> Add1/2
  Unit Delay1/1 -> Add1/1
  Add1/1 -> Display/1, Unit Delay1/1, Scope/1
  Switch/1 -> Unit Delay/1, Scope1/1, Relational Operator1/1
  Unit Delay/1 -> Add/1
  In1/1 -> Data Type Conversion2/1
  Add/1 -> Switch/1
  Saturation/1 -> Add2/1

== system EPT/Foreground_TimeBase_5ms/Oil//Water//Pack Cooling System/AirC1/Delay5/CycleTrigger ==
  In1 : Inport
  In2 : Inport  Port=2
  Add : Sum
  Add1 : Sum
  Add2 : Sum  Inputs=+-
  Constant1 : Constant
  Constant2 : Constant  Value=0
  Constant3 : Constant
  Data Type Conversion1 : DataTypeConversion
  Data Type Conversion2 : DataTypeConversion
  Display : Display
  Relational Operator1 : RelationalOperator  OutDataTypeStr=boolean  RndMeth=Simplest
  Saturation : Saturate  UpperLimit=inf  LowerLimit=2
  Scope : Scope
  Scope1 : Scope
  Scope2 : Scope
  Switch : Switch  Threshold=1
  Unit Delay : UnitDelay  SampleTime=-1  HasFrameUpgradeWarning=on
  Unit Delay1 : UnitDelay  SampleTime=-1  HasFrameUpgradeWarning=on
  Trigger : Outport  VectorParamsAs1DForOutWhenUnconnected=off
  wires:
  Constant3/1 -> Add2/2
  In2/1 -> Saturation/1
  Add2/1 -> Data Type Conversion1/1
  Data Type Conversion2/1 -> Switch/2, Add/2
  Constant2/1 -> Switch/3
  Data Type Conversion1/1 -> Relational Operator1/2
  Relational Operator1/1 -> Trigger/1, Scope2/1
  Constant1/1 -> Add1/2
  Unit Delay1/1 -> Add1/1
  Add1/1 -> Display/1, Unit Delay1/1, Scope/1
  Switch/1 -> Unit Delay/1, Scope1/1, Relational Operator1/1
  Unit Delay/1 -> Add/1
  In1/1 -> Data Type Conversion2/1
  Add/1 -> Switch/1
  Saturation/1 -> Add2/1

== system EPT/Foreground_TimeBase_5ms/Oil//Water//Pack Cooling System/AirC1/Delay6/CycleTrigger ==
  In1 : Inport
  In2 : Inport  Port=2
  Add : Sum
  Add1 : Sum
  Add2 : Sum  Inputs=+-
  Constant1 : Constant
  Constant2 : Constant  Value=0
  Constant3 : Constant
  Data Type Conversion1 : DataTypeConversion
  Data Type Conversion2 : DataTypeConversion
  Display : Display
  Relational Operator1 : RelationalOperator  OutDataTypeStr=boolean  RndMeth=Simplest
  Saturation : Saturate  UpperLimit=inf  LowerLimit=2
  Scope : Scope
  Scope1 : Scope
  Scope2 : Scope
  Switch : Switch  Threshold=1
  Unit Delay : UnitDelay  SampleTime=-1  HasFrameUpgradeWarning=on
  Unit Delay1 : UnitDelay  SampleTime=-1  HasFrameUpgradeWarning=on
  Trigger : Outport  VectorParamsAs1DForOutWhenUnconnected=off
  wires:
  Constant3/1 -> Add2/2
  In2/1 -> Saturation/1
  Add2/1 -> Data Type Conversion1/1
  Data Type Conversion2/1 -> Switch/2, Add/2
  Constant2/1 -> Switch/3
  Data Type Conversion1/1 -> Relational Operator1/2
  Relational Operator1/1 -> Trigger/1, Scope2/1
  Constant1/1 -> Add1/2
  Unit Delay1/1 -> Add1/1
  Add1/1 -> Display/1, Unit Delay1/1, Scope/1
  Switch/1 -> Unit Delay/1, Scope1/1, Relational Operator1/1
  Unit Delay/1 -> Add/1
  In1/1 -> Data Type Conversion2/1
  Add/1 -> Switch/1
  Saturation/1 -> Add2/1

== system EPT/Foreground_TimeBase_5ms/Oil//Water//Pack Cooling System/AirC1/Delay7/CycleTrigger ==
  In1 : Inport
  In2 : Inport  Port=2
  Add : Sum
  Add1 : Sum
  Add2 : Sum  Inputs=+-
  Constant1 : Constant
  Constant2 : Constant  Value=0
  Constant3 : Constant
  Data Type Conversion1 : DataTypeConversion
  Data Type Conversion2 : DataTypeConversion
  Display : Display
  Relational Operator1 : RelationalOperator  OutDataTypeStr=boolean  RndMeth=Simplest
  Saturation : Saturate  UpperLimit=inf  LowerLimit=2
  Scope : Scope
  Scope1 : Scope
  Scope2 : Scope
  Switch : Switch  Threshold=1
  Unit Delay : UnitDelay  SampleTime=-1  HasFrameUpgradeWarning=on
  Unit Delay1 : UnitDelay  SampleTime=-1  HasFrameUpgradeWarning=on
  Trigger : Outport  VectorParamsAs1DForOutWhenUnconnected=off
  wires:
  Constant3/1 -> Add2/2
  In2/1 -> Saturation/1
  Add2/1 -> Data Type Conversion1/1
  Data Type Conversion2/1 -> Switch/2, Add/2
  Constant2/1 -> Switch/3
  Data Type Conversion1/1 -> Relational Operator1/2
  Relational Operator1/1 -> Trigger/1, Scope2/1
  Constant1/1 -> Add1/2
  Unit Delay1/1 -> Add1/1
  Add1/1 -> Display/1, Unit Delay1/1, Scope/1
  Switch/1 -> Unit Delay/1, Scope1/1, Relational Operator1/1
  Unit Delay/1 -> Add/1
  In1/1 -> Data Type Conversion2/1
  Add/1 -> Switch/1
  Saturation/1 -> Add2/1

== system EPT/Foreground_TimeBase_5ms/System Setup/Dyno_Test /Dyno Test/Latch ==
  Latch : Inport
  Reset : Inport  Port=2
  Switch1 : Switch  Criteria=u2 > Threshold
  Switch3 : Switch  Criteria=u2 > Threshold
  Unit Delay1 : UnitDelay  SampleTime=-1  HasFrameUpgradeWarning=on
  Output : Outport  VectorParamsAs1DForOutWhenUnconnected=off
  wires:
  Unit Delay1/1 -> Switch1/3
  Switch3/1 -> Output/1, Unit Delay1/1
  Reset/1 -> Switch3/2
  Latch/1 -> Switch1/1, Switch1/2
  Switch1/1 -> Switch3/3

== system EPT/Foreground_TimeBase_5ms/System Setup/Dyno_Test /Dyno Test/MCU Tq MAP_Inc ==
  Enable : Inport
  Tq_Max : Inport  Port=2
  Torque_Inc_unit : Inport  Port=3
  AND : Logic  IconShape=distinctive  AllPortsSameDT=off  OutDataTypeStr=boolean
  Abs : Abs
  Abs1 : Abs
  Add : Sum
  Gain : Gain  Gain=-1
  Product : Product
  Relational Operator : RelationalOperator  Operator=>  OutDataTypeStr=boolean  RndMeth=Simplest
  Relational Operator1 : RelationalOperator  Operator===  OutDataTypeStr=boolean  RndMeth=Simplest
  Saturation Dynamic : simulink/Discontinuities/Saturation Dynamic  OutMin=[]  OutMax=[]  OutDataTypeStr=Inherit: Same as second input  OutDataType=fixdt(1, 16)  OutScaling=2^-10  DoSatur=off
  Scope : Scope
  Switch1 : Switch  Criteria=u2 > Threshold
  Unit Delay : UnitDelay  SampleTime=-1  HasFrameUpgradeWarning=on
  Command_Tq : Outport  VectorParamsAs1DForOutWhenUnconnected=off
  Flag : Outport  Port=2  VectorParamsAs1DForOutWhenUnconnected=off
  wires:
  Torque_Inc_unit/1 -> Product/1, Add/1
  Unit Delay/1 -> Command_Tq/1, Scope/1, Relational Operator1/1, Add/2
  Tq_Max/1 -> Relational Operator1/2, Product/2, Abs1/1, Abs/1
  Switch1/1 -> Unit Delay/1
  Saturation Dynamic/1 -> Switch1/1
  Abs1/1 -> Gain/1
  Abs/1 -> Saturation Dynamic/1
  Add/1 -> Saturation Dynamic/2
  Gain/1 -> Saturation Dynamic/3
  Enable/1 -> AND/1
  AND/1 -> Switch1/2
  Product/1 -> Relational Operator/1
  Relational Operator/1 -> AND/2
  Relational Operator1/1 -> Flag/1

== system EPT/Foreground_TimeBase_5ms/System Setup/Dyno_Test /Dyno Test/MCU Tq MAP_Manual ==
  Enable : Inport
  Tq_Max : Inport  Port=2
  Target_Torque_Manual : Inport  Port=3
  Abs : Abs
  Abs1 : Abs
  Gain : Gain  Gain=-1
  Saturation Dynamic : simulink/Discontinuities/Saturation Dynamic  OutMin=[]  OutMax=[]  OutDataTypeStr=Inherit: Same as second input  OutDataType=fixdt(1, 16)  OutScaling=2^-10  DoSatur=off
  Switch1 : Switch  Criteria=u2 > Threshold
  Command_Tq : Outport  VectorParamsAs1DForOutWhenUnconnected=off
  wires:
  Saturation Dynamic/1 -> Switch1/1
  Enable/1 -> Switch1/2
  Target_Torque_Manual/1 -> Saturation Dynamic/2
  Abs/1 -> Saturation Dynamic/1
  Abs1/1 -> Gain/1
  Gain/1 -> Saturation Dynamic/3
  Tq_Max/1 -> Abs1/1, Abs/1
  Switch1/1 -> Command_Tq/1

== system EPT/Foreground_TimeBase_5ms/System Setup/HV_Setup()/CHG_Mode/CHG Full Flag ==
  Delay : Subsystem
  Gain : Gain  Gain=200
  Latch2 : Subsystem
  Relational Operator : RelationalOperator  OutDataTypeStr=boolean  RndMeth=Simplest
  raptor_adjustment : Raptor_lib/Data Storage/raptor_adjustment  paramName='CHG_SOC_Limit'  nameSource=Parameter  initValue=75  dataType=double  storage=Calibration  calDispType=Number  calEnum={'False', 'True'}  calGain=1.0  calOffset=0.0  calMax=inf  calMin=-inf  calFormat='-1'  calUnit=''  calHelp=''  calAccess=1  calFunction=raptor_xcp_function(gcb)  calDispHeaders=off  calColHeaders={'Col1' 'Col2' 'Col3'}  calRowHeaders={'Row1' 'Row2' 'Row3'}
      settings: SourceProductName=Raptor
  raptor_adjustment1 : Raptor_lib/Data Storage/raptor_adjustment  paramName='Delay_CHG_Full'  nameSource=Parameter  initValue=30  dataType=double  storage=Calibration  calDispType=Number  calEnum={'False', 'True'}  calGain=1.0  calOffset=0.0  calMax=inf  calMin=-inf  calFormat='-1'  calUnit=''  calHelp=''  calAccess=1  calFunction=raptor_xcp_function(gcb)  calDispHeaders=off  calColHeaders={'Col1' 'Col2' 'Col3'}  calRowHeaders={'Row1' 'Row2' 'Row3'}
      settings: SourceProductName=Raptor
  raptor_adjustment2 : Raptor_lib/Data Storage/raptor_adjustment  paramName='Reset_CHG_Full_Flag'  nameSource=Parameter  initValue=0  dataType=double  storage=Calibration  calDispType=Number  calEnum={'False', 'True'}  calGain=1.0  calOffset=0.0  calMax=inf  calMin=-inf  calFormat='-1'  calUnit=''  calHelp=''  calAccess=1  calFunction=raptor_xcp_function(gcb)  calDispHeaders=off  calColHeaders={'Col1' 'Col2' 'Col3'}  calRowHeaders={'Row1' 'Row2' 'Row3'}
      settings: SourceProductName=Raptor
  raptor_data_read14 : Raptor_lib/Data Storage/raptor_data_read  dataName='Fault_Reset_Trigger'  dataShape=Scalar  idxSource=Input  idxRow=1  idxCol=1
      settings: SourceProductName=Raptor
  Out1 : Outport  VectorParamsAs1DForOutWhenUnconnected=off
  wires:
  raptor_adjustment1/1 -> Gain/1
  Gain/1 -> Delay/2(TimeCount)
  raptor_adjustment/1 -> Relational Operator/2
  Delay/1(Output) -> Latch2/1(Latch)
  raptor_adjustment2/1 -> Latch2/2(Reset)
  Relational Operator/1 -> Delay/1(Condition)
  Latch2/1(Output) -> Out1/1
  raptor_data_read14/1 -> Relational Operator/1
